simulink model "land_V0"  (R2023b)
settings: Solver=ode4  StartTime=0.0  StopTime=150  FixedStep=0.001  RelTol=1e-3
values from neighbouring files (symbols this model uses):
  a0 = 340.294    [basedata.m]    (also in basedata.mat; control_design.mat; landing_init.m; landing_plan.mat)
  b_ref = 2.0    (= 2)    [basedata.m]    (also in basedata.mat; control_design.mat; landing_init.m; landing_plan.mat)
  c_gear = [0.8e4, 1.4e4, 1.4e4]    [basedata.m]    (also in basedata.mat = [8000 14000 14000]; control_design.mat = [8000 14000 14000]; landing_init.m; landing_plan.mat = [8000 14000 14000])
  c_lat = [1.4e4, 2.2e4, 2.2e4]    [basedata.m]    (also in basedata.mat = [14000 22000 22000]; control_design.mat = [14000 22000 22000]; landing_init.m; landing_plan.mat = [14000 22000 22000])
  c_ref = 0.9    [basedata.m]    (also in basedata.mat; control_design.mat; landing_init.m; landing_plan.mat)
  c_roll = [0.020, 0.018, 0.018]    [basedata.m]    (also in basedata.mat = [0.02 0.018 0.018]; control_design.mat = [0.02 0.018 0.018]; landing_init.m; landing_plan.mat = [0.02 0.018 0.018])
  CD0 = 0.045    [basedata.m]    (also in basedata.mat; canshujisuan.m; control_design.mat; landing_init.m)
  CL0 = 0.083    [basedata.m]    (also in basedata.mat; control_design.mat; landing_init.m; landing_plan.mat)
  CLa = 3.80    (= 3.8)    [basedata.m]    (also in basedata.mat; canshujisuan.m = 2.5; control_design.mat; landing_init.m)
  Clb = -0.08    [basedata.m]    (also in basedata.mat; control_design.mat; landing_init.m; landing_plan.mat)
  Clda = -0.20    (= -0.2)    [basedata.m]    (also in basedata.mat; control_design.mat; landing_init.m; landing_plan.mat)
  CLde = 0.28    [basedata.m]    (also in basedata.mat; control_design.mat; landing_init.m; landing_plan.mat)
  Clp = -0.70    (= -0.7)    [basedata.m]    (also in basedata.mat; control_design.mat; landing_init.m; landing_plan.mat)
  CLq = 4.50    (= 4.5)    [basedata.m]    (also in basedata.mat; canshujisuan.m = 3; control_design.mat; landing_init.m)
  Clr = 0.08    [basedata.m]    (also in basedata.mat; control_design.mat; landing_init.m; landing_plan.mat)
  Cm0 = 0.060    (= 0.06)    [basedata.m]    (also in basedata.mat; control_design.mat; landing_init.m; landing_plan.mat)
  Cma = -0.80    (= -0.8)    [basedata.m]    (also in basedata.mat; control_design.mat; landing_init.m; landing_plan.mat)
  Cmde = -0.90    (= -0.9)    [basedata.m]    (also in basedata.mat; control_design.mat; landing_init.m; landing_plan.mat)
  Cmq = -18.0    (= -18)    [basedata.m]    (also in basedata.mat; control_design.mat; landing_init.m; landing_plan.mat)
  Cnb = 0.25    [basedata.m]    (also in basedata.mat; control_design.mat; landing_init.m; landing_plan.mat)
  Cndr = -0.15    [basedata.m]    (also in basedata.mat; control_design.mat; landing_init.m; landing_plan.mat)
  Cnp = -0.04    [basedata.m]    (also in basedata.mat; control_design.mat; landing_init.m; landing_plan.mat)
  Cnr = -0.45    [basedata.m]    (also in basedata.mat; control_design.mat; landing_init.m; landing_plan.mat)
  CSb = -0.70    (= -0.7)    [basedata.m]    (also in basedata.mat; control_design.mat; landing_init.m; landing_plan.mat)
  CSdr = 0.18    [basedata.m]    (also in basedata.mat; control_design.mat; landing_init.m; landing_plan.mat)
  CSr = 0.12    [basedata.m]    (also in basedata.mat; control_design.mat; landing_init.m; landing_plan.mat)
  D = 0.5 * rho0 * V^2 * S_ref * CD_current    [canshujisuan.m]
  D0 = 1400    [basedata.m]    (also in basedata.mat; control_design.mat = 800; landing.m; landing_init.m)
  da_max = 25    [basedata.m]    (also in basedata.mat; control_design.mat; landing_init.m; landing_plan.mat)
  da_min = -da_max    (= -25)    [basedata.m]    (also in basedata.mat; control_design.mat; landing_init.m; landing_plan.mat)
  de_max = 25    [basedata.m]    (also in basedata.mat; control_design.mat; landing_init.m; landing_plan.mat)
  de_min = -de_max    (= -25)    [basedata.m]    (also in basedata.mat; control_design.mat; landing_init.m; landing_plan.mat)
  DH = pi / 180    (= 0.0174532925199)    [basedata.m]    (also in basedata.mat; control_design.mat; landing_init.m; landing_plan.mat)
  dr_max = 25    [basedata.m]    (also in basedata.mat; control_design.mat; landing_init.m; landing_plan.mat)
  dr_min = -dr_max    (= -25)    [basedata.m]    (also in basedata.mat; control_design.mat; landing_init.m; landing_plan.mat)
  g = 9.80665    [basedata.m]    (also in basedata.mat; canshujisuan.m; control_design.mat; landing_init.m)
  gamma1 = -0.125844364415    [basedata.mat]    (also in landing_trajectory.m = asin(max(min(gamma1_arg, 1), -1)); landingplan.mat)
  gamma2 = -0.0261780104712    [basedata.mat]    (also in landing_trajectory.m = -0.0261799387799; landingplan.mat = 0.0261780104712)
  ground_z = 0.0    (= 0)    [basedata.m]    (also in basedata.mat; control_design.mat; landing_init.m; landing_plan.mat)
  HD = 180 / pi    (= 57.2957795131)    [basedata.m]    (also in basedata.mat; control_design.mat; landing_init.m; landing_plan.mat)
  I = [ Ixx, -Ixy, -Ixz ... (first row only)    [basedata.m]    (also in basedata.mat = [120  0  0; 0  480  0; 0  0  520]; control_design.mat = [120  0  0; 0  480  0; 0  0  520]; landing_init.m; landing_plan.mat = [120  0  0; 0  480  0; 0  0  520])
  K = 0.12    [basedata.m]    (also in basedata.mat; canshujisuan.m = 0.08; control_design.mat; landing_init.m)
  K_alpha = 7.5375    [basedata.mat]    (also in control_design.m = (((wd_pitch^2)-a24))/(2*kesi_pitch*wd_pitch); control_design.mat; controller.m = 5; landingplan.mat)
  k_gear = [1.0e5, 3.0e5, 3.0e5]    [basedata.m]    (also in basedata.mat = [100000 300000 300000]; control_design.mat = [100000 300000 300000]; landing_init.m; landing_plan.mat = [100000 300000 300000])
  Kn_pitch = -0.120095403309    [basedata.mat]    (also in control_design.m = -(2.2*g*(wd_pitch)^2)/(Tr*(((wd_pitch)^2)-a24)*V_control*a34; control_design.mat; controller.m = (2.2*wd^2*g)/(Tr*(wd^2-a24)*V_test*a34); landingplan.mat)
  Kw_pitch = -0.483749055178    [basedata.mat]    (also in control_design.m = -2*kesi_pitch*wd_pitch/a25; control_design.mat; controller.m = -(2*zeta*wd) / a25; landingplan.mat)
  m = 600.0    (= 600)    [basedata.m]    (also in basedata.mat; canshujisuan.m; control_design.mat; landing_init.m)
  mu_brake = [0.0, 0.55, 0.55]    [basedata.m]    (also in basedata.mat = [0 0.55 0.55]; control_design.mat = [0 0.55 0.55]; landing_init.m; landing_plan.mat = [0 0.55 0.55])
  phi0 = 0    [control_design.mat]    (also in landing.m; landing_init.m; landing_init.mat; landing_plan.mat)
  psi0 = 0    [control_design.mat]    (also in landing.m; landing_init.m; landing_init.mat; landing_plan.mat)
  r_left_b = r_gear_b(:,2)    [basedata.m]    (also in basedata.mat = [-0.333333333333 -0.8 0.65]; control_design.mat = [-0.333333333333 -0.8 0.65]; landing_init.m; landing_plan.mat = [-0.333333333333 -0.8 0.65])
  r_nose_b = r_gear_b(:,1)    [basedata.m]    (also in basedata.mat = [2 0 0.65]; control_design.mat = [2 0 0.65]; landing_init.m; landing_plan.mat = [2 0 0.65])
  r_right_b = r_gear_b(:,3)    [basedata.m]    (also in basedata.mat = [-0.333333333333 0.8 0.65]; control_design.mat = [-0.333333333333 0.8 0.65]; landing_init.m; landing_plan.mat = [-0.333333333333 0.8 0.65])
  rho0 = 1.225    [basedata.m]    (also in basedata.mat; canshujisuan.m; control_design.mat; landing_init.m)
  S_ref = 1.2    [basedata.m]    (also in basedata.mat; canshujisuan.m; control_design.mat; landing_init.m)
  theta0 = 0    [control_design.mat]    (also in landing.m; landing_init.m; landing_init.mat = 0.0523598775598; landing_plan.mat = 0.0523560209424)
  u0_b = 0    [control_design.mat]    (also in landing.m = 128; landing_init.m = 128; landing_init.mat = 100; landing_plan.mat = 128)
  v0_b = 0    [control_design.mat]    (also in landing.m; landing_init.m; landing_init.mat; landing_plan.mat)
  v_eps = 0.20    (= 0.2)    [basedata.m]    (also in basedata.mat; control_design.mat; landing_init.m; landing_plan.mat)
  V_min = 3    [control_design.mat]    (also in landing.m; landing_init.m; landing_plan.mat; landingplan.mat)
  w0_b = 0    [control_design.mat]    (also in landing.m; landing_init.m; landing_init.mat; landing_plan.mat)
  wheel_radius = 0.18    [basedata.m]    (also in basedata.mat; control_design.mat; landing_init.m; landing_plan.mat)
  WOW_on = 0.000    (= 0)    [basedata.m]    (also in basedata.mat; control_design.mat; landing_init.m; landing_plan.mat)
  Xg0 = 0    [control_design.mat]    (also in landing.m = -12000; landing_init.m = -12000; landing_init.mat = -8000; landing_plan.mat = -12000)
  Yg0 = 3    [control_design.mat]    (also in landing.m = 0; landing_init.m = 0; landing_init.mat = 0; landing_plan.mat = 0)
  Zg0 = ground_z - wheel_radius - r_gear_b(3,1) + static_deflection    [basedata.m]    (also in basedata.mat = -0.8215943; control_design.mat = -0.8215943; landing.m = -1000; landing_init.m = -1000)
undefined symbols (not defined in the file or in its folder): I_xz, I_yz, Ix_Iy, Iy_Iz, Iz_Ix
libraries: simulink x37, matrix_library x19
(part 3 of 3)

== system land_V0/6DOF-MODEL/动力学/起落架模型/起落架三轮质心在地系下位置 ==
  Add : Sum
  Add1 : Sum
  Add2 : Sum
  Constant : Constant  Value=r_nose_b
  Constant1 : Constant  Value=r_left_b
  Constant2 : Constant  Value=r_right_b
  MATLAB Function : MATLAB Function  TreatAsAtomicUnit=on
  Matrix Multiply : Product  Multiplication=Matrix(*)
  Matrix Multiply1 : Product  Multiplication=Matrix(*)
  Matrix Multiply2 : Product  Multiplication=Matrix(*)
  Mux : Mux  Inputs=3
  Scope : Scope
  Scope1 : Scope
  Scope2 : Scope
  Selector : Selector  InputPortWidth=3  IndexOptions=Index vector (dialog)  Indices=2  OutputSizes=1
  Transpose : matrix_library/Transpose
  Nose_pos_g : Outport
  Left_pos_g : Outport  Port=2
  Right_pos_g : Outport  Port=3
  tag scope: Left_pos_g=global, Nose_position_g=global, Right_pos_g=global
  wires:
  Constant1/1 -> Matrix Multiply1/2
  Transpose/1 -> Matrix Multiply2/1, Matrix Multiply1/1, Matrix Multiply/1
  [psi_eular] -> MATLAB Function/3(psi)
  [phi_eular] -> MATLAB Function/1(phi), Scope2/1
  Constant2/1 -> Matrix Multiply2/2
  Matrix Multiply1/1 -> Add1/2
  Constant/1 -> Matrix Multiply/2
  [theta_eular] -> MATLAB Function/2(theta)
  MATLAB Function/1(R_bg) -> Transpose/1
  Matrix Multiply/1 -> Add/2
  Matrix Multiply2/1 -> Add2/2
  [Z_positon] -> Mux/3
  [Y_positon] -> Scope1/1, Mux/2
  [X_positon] -> Mux/1
  Mux/1 -> Add/1, Add1/1, Add2/1
  Add/1 -> Selector/1, Nose_pos_g/1, [Nose_position_g]
  Add1/1 -> Left_pos_g/1, [Left_pos_g]
  Add2/1 -> Right_pos_g/1, [Right_pos_g]
  Selector/1 -> Scope/1

== system land_V0/6DOF-MODEL/动力学/起落架模型/轮胎压缩量计算 ==
  Nose_pos_g : Inport
  Left_pos_g : Inport  Port=2
  Right_pos_g : Inport  Port=3
  Constant : Constant  Value=wheel_radius
  Constant1 : Constant  Value=ground_z
  Constant2 : Constant  Value=0
  Constant4 : Constant
  Saturation : Saturate  UpperLimit=wheel_radius  LowerLimit=0
  Saturation1 : Saturate  UpperLimit=wheel_radius  LowerLimit=0
  Saturation2 : Saturate  UpperLimit=wheel_radius  LowerLimit=0
  Scope : Scope
  Scope1 : Scope
  Selector : Selector  InputPortWidth=3  IndexOptions=Index vector (dialog)  Indices=3  OutputSizes=1
  Selector1 : Selector  InputPortWidth=3  IndexOptions=Index vector (dialog)  Indices=3  OutputSizes=1
  Selector2 : Selector  InputPortWidth=3  IndexOptions=Index vector (dialog)  Indices=3  OutputSizes=1
  Subtract{,1..5} (6 alike) : Sum  Inputs=+-
  Switch3 : Switch  Criteria=u2 > Threshold  Threshold=WOW_on  SaturateOnIntegerOverflow=off  InputSameDT=off
  Switch4 : Switch  Criteria=u2 > Threshold  Threshold=WOW_on  SaturateOnIntegerOverflow=off  InputSameDT=off
  Switch5 : Switch  Criteria=u2 > Threshold  Threshold=WOW_on  SaturateOnIntegerOverflow=off  InputSameDT=off
  delta_nose : Outport
  delta_left : Outport  Port=2
  delta_right : Outport  Port=3
  tag scope: contact_left=global, contact_nose=global, contact_right=global, delta_left=global, delta_nose=global, delta_right=global
  wires:
  Nose_pos_g/1 -> Selector/1
  Left_pos_g/1 -> Selector1/1
  Right_pos_g/1 -> Selector2/1
  Subtract/1 -> Subtract3/2
  Subtract1/1 -> Subtract4/2
  Subtract2/1 -> Subtract5/2
  Constant/1 -> Subtract5/1, Subtract4/1, Subtract3/1
  Saturation/1 -> Scope/1, delta_nose/1, [delta_nose]
  Saturation1/1 -> [delta_left], delta_left/1, Scope1/1
  Saturation2/1 -> [delta_right], delta_right/1
  Subtract3/1 -> Switch3/2, Saturation/1
  Subtract4/1 -> Switch4/2, Saturation1/1
  Subtract5/1 -> Switch5/2, Saturation2/1
  Constant2/1 -> Switch3/3, Switch5/3, Switch4/3
  Constant4/1 -> Switch5/1, Switch4/1, Switch3/1
  Switch3/1 -> [contact_nose]
  Switch5/1 -> [contact_right]
  Switch4/1 -> [contact_left]
  Constant1/1 -> Subtract/1, Subtract1/1, Subtract2/1
  Selector/1 -> Subtract/2
  Selector1/1 -> Subtract1/2
  Selector2/1 -> Subtract2/2

== system land_V0/controller1/1_Pitch_Ctrl/567三回路控制/Subsystem ==
  q : Inport
  Integrator : Integrator
  Product : Product
  Subsystem : Subsystem
  Sum : Sum  Inputs=|+-
  alpha(伪攻角) : Outport
  wires:
  q/1 -> Sum/1
  Sum/1 -> Integrator/1
  Integrator/1 -> Product/1, alpha(伪攻角)/1
  Product/1 -> Sum/2
  Subsystem/1(a34) -> Product/2

== system land_V0/6DOF-MODEL/动力学/起落架模型/三轮在地系下的力/摩擦圆限幅 ==
  N_nose : Inport
  N_left : Inport  Port=2
  N_right : Inport  Port=3
  F_long_nose : Inport  Port=4
  F_long_left : Inport  Port=5
  F_long_right : Inport  Port=6
  F_lat_nose : Inport  Port=7
  F_lat_left : Inport  Port=8
  F_lat_right : Inport  Port=9
  主轮摩擦圆限幅右 : MATLAB Function  TreatAsAtomicUnit=on
  主轮摩擦圆限幅左 : MATLAB Function  TreatAsAtomicUnit=on
  前轮摩擦圆限幅 : MATLAB Function  TreatAsAtomicUnit=on
  F_long_nose_out : Outport
  F_long_left_out : Outport  Port=2
  F_long_right_out : Outport  Port=3
  F_lat__nose_out : Outport  Port=4
  F_lat_left_out : Outport  Port=5
  F_lat_right_out : Outport  Port=6
  wires:
  前轮摩擦圆限幅/1(F_long_out) -> F_long_nose_out/1
  前轮摩擦圆限幅/2(F_lat_out) -> F_lat__nose_out/1
  主轮摩擦圆限幅左/2(F_lat_out) -> F_lat_left_out/1
  主轮摩擦圆限幅左/1(F_long_out) -> F_long_left_out/1
  主轮摩擦圆限幅右/2(F_lat_out) -> F_lat_right_out/1
  主轮摩擦圆限幅右/1(F_long_out) -> F_long_right_out/1
  N_nose/1 -> 前轮摩擦圆限幅/1(N)
  F_long_nose/1 -> 前轮摩擦圆限幅/2(F_long)
  F_lat_nose/1 -> 前轮摩擦圆限幅/3(F_lat)
  F_long_left/1 -> 主轮摩擦圆限幅左/2(F_long)
  N_left/1 -> 主轮摩擦圆限幅左/1(N)
  F_lat_right/1 -> 主轮摩擦圆限幅右/3(F_lat)
  F_lat_left/1 -> 主轮摩擦圆限幅左/3(F_lat)
  F_long_right/1 -> 主轮摩擦圆限幅右/2(F_long)
  N_right/1 -> 主轮摩擦圆限幅右/1(N)

== system land_V0/6DOF-MODEL/动力学/起落架模型/侧向力/Subsystem ==
  delt-s(H) : Inport
  Constant : Constant  Value=0
  Constant1 : Constant  Value=0
  Constant2 : Constant  Value=0
  Constant3 : Constant
  Cos : Trigonometry  Operator=cos
  Gain : Gain  Gain=-1
  Hermitian Transpose{,1..3} (4 alike) : matrix_library/Hermitian Transpose
  MATLAB Function : MATLAB Function  TreatAsAtomicUnit=on
  Matrix Multiply : Product  Multiplication=Matrix(*)
  Matrix Multiply1 : Product  Multiplication=Matrix(*)
  Matrix Multiply2 : Product  Multiplication=Matrix(*)
  Mux : Mux  Inputs=3
  Mux1 : Mux  Inputs=3
  Reshape : Reshape  OutputDimensionality=Column vector (2-D)
  Reshape1 : Reshape  OutputDimensionality=Column vector (2-D)
  Sin : Trigonometry
  主轮侧向方向向量 : MATLAB Function  TreatAsAtomicUnit=on
  前轮侧向向量 : MATLAB Function  TreatAsAtomicUnit=on
  V_lat_nose : Outport
  V_lat_left : Outport  Port=2
  V_lat_right : Outport  Port=3
  tag scope: V_lat_left=global, V_lat_nose=global, V_lat_right=global, e_g_lat_main=global, e_g_lat_nose=global
  wires:
  MATLAB Function/1(R_bg) -> Hermitian Transpose/1
  [phi_eular] -> MATLAB Function/1(phi)
  Hermitian Transpose/1 -> 主轮侧向方向向量/1(Cbg), 前轮侧向向量/1(Cbg)
  Mux/1 -> Reshape/1
  Constant1/1 -> Mux1/1
  Mux1/1 -> Reshape1/1
  [V_nose_g] -> Hermitian Transpose1/1
  前轮侧向向量/1(eg_lat) -> [e_g_lat_nose], Matrix Multiply/2
  Hermitian Transpose1/1 -> Matrix Multiply/1
  [V_left_g] -> Hermitian Transpose2/1
  [V_right_g] -> Hermitian Transpose3/1
  主轮侧向方向向量/1(eg_lat) -> Matrix Multiply2/2, Matrix Multiply1/2, [e_g_lat_main]
  Hermitian Transpose3/1 -> Matrix Multiply1/1
  Hermitian Transpose2/1 -> Matrix Multiply2/1
  Matrix Multiply/1 -> V_lat_nose/1, [V_lat_nose]
  Matrix Multiply2/1 -> V_lat_left/1, [V_lat_left]
  Matrix Multiply1/1 -> V_lat_right/1, [V_lat_right]
  Sin/1 -> Gain/1
  Gain/1 -> Mux/1
  delt-s(H)/1 -> Sin/1, Cos/1
  [theta_eular] -> MATLAB Function/2(theta)
  [psi_eular] -> MATLAB Function/3(psi)
  Reshape/1 -> 前轮侧向向量/2(eb_lat)
  Reshape1/1 -> 主轮侧向方向向量/2(eb_lat)
  Cos/1 -> Mux/2
  Constant/1 -> Mux/3
  Constant3/1 -> Mux1/2
  Constant2/1 -> Mux1/3

== system land_V0/6DOF-MODEL/动力学/起落架模型/侧向力/Subsystem1 ==
  In1 : Inport
  Constant5 : Constant  Value=0
  Switch : Switch  Criteria=u2 > Threshold  SaturateOnIntegerOverflow=off  InputSameDT=off
  F_lat_left : Outport
  wires:
  In1/1 -> Switch/1
  Constant5/1 -> Switch/3
  Switch/1 -> F_lat_left/1
  [contact_left] -> Switch/2

== system land_V0/6DOF-MODEL/动力学/起落架模型/侧向力/Subsystem2 ==
  In1 : Inport
  Constant5 : Constant  Value=0
  Switch : Switch  Criteria=u2 > Threshold  SaturateOnIntegerOverflow=off  InputSameDT=off
  F_lat_nose : Outport
  wires:
  In1/1 -> Switch/1
  Constant5/1 -> Switch/3
  Switch/1 -> F_lat_nose/1
  [contact_nose] -> Switch/2

== system land_V0/6DOF-MODEL/动力学/起落架模型/侧向力/Subsystem3 ==
  In1 : Inport
  Constant5 : Constant  Value=0
  Switch : Switch  Criteria=u2 > Threshold  SaturateOnIntegerOverflow=off  InputSameDT=off
  F_lat_right : Outport
  wires:
  [contact_right] -> Switch/2
  Switch/1 -> F_lat_right/1
  Constant5/1 -> Switch/3
  In1/1 -> Switch/1

== system land_V0/6DOF-MODEL/动力学/起落架模型/法向支反力/Subsystem ==
  In1 : Inport
  Constant5 : Constant  Value=0
  Switch : Switch  Criteria=u2 > Threshold  SaturateOnIntegerOverflow=off  InputSameDT=off
  N_nose : Outport
  wires:
  In1/1 -> Switch/1
  Constant5/1 -> Switch/3
  Switch/1 -> N_nose/1
  [contact_nose] -> Switch/2

== system land_V0/6DOF-MODEL/动力学/起落架模型/法向支反力/Subsystem1 ==
  In1 : Inport
  Constant5 : Constant  Value=0
  Switch : Switch  Criteria=u2 > Threshold  SaturateOnIntegerOverflow=off  InputSameDT=off
  N_left : Outport
  wires:
  [contact_left] -> Switch/2
  Switch/1 -> N_left/1
  Constant5/1 -> Switch/3
  In1/1 -> Switch/1

== system land_V0/6DOF-MODEL/动力学/起落架模型/法向支反力/Subsystem2 ==
  In1 : Inport
  Constant5 : Constant  Value=0
  Switch : Switch  Criteria=u2 > Threshold  SaturateOnIntegerOverflow=off  InputSameDT=off
  N_right : Outport
  wires:
  In1/1 -> Switch/1
  Constant5/1 -> Switch/3
  Switch/1 -> N_right/1
  [contact_right] -> Switch/2

== system land_V0/6DOF-MODEL/动力学/起落架模型/纵向力/Subsystem ==
  delt-s(H) : Inport
  Constant : Constant  Value=0
  Constant1 : Constant
  Constant2 : Constant  Value=0
  Constant3 : Constant  Value=0
  Cos : Trigonometry  Operator=cos
  Hermitian Transpose{,1..3} (4 alike) : matrix_library/Hermitian Transpose
  MATLAB Function : MATLAB Function  TreatAsAtomicUnit=on
  Matrix Multiply : Product  Multiplication=Matrix(*)
  Matrix Multiply1 : Product  Multiplication=Matrix(*)
  Matrix Multiply2 : Product  Multiplication=Matrix(*)
  Mux : Mux  Inputs=3
  Mux1 : Mux  Inputs=3
  Reshape : Reshape  OutputDimensionality=Column vector (2-D)
  Reshape1 : Reshape  OutputDimensionality=Column vector (2-D)
  Sin : Trigonometry
  主轮滚动方向向量 : MATLAB Function  TreatAsAtomicUnit=on
  前轮滚动方向向量 : MATLAB Function  TreatAsAtomicUnit=on
  V_long_nose : Outport
  V_long_left : Outport  Port=2
  V_long_right : Outport  Port=3
  tag scope: V_long_left=global, V_long_nose=global, V_long_right=global, e_g_long_main=global, e_g_long_nose=global
  wires:
  MATLAB Function/1(R_bg) -> Hermitian Transpose/1
  [phi_eular] -> MATLAB Function/1(phi)
  Hermitian Transpose/1 -> 主轮滚动方向向量/1(Cbg), 前轮滚动方向向量/1(Cbg)
  delt-s(H)/1 -> Cos/1, Sin/1
  Cos/1 -> Mux/1
  Mux/1 -> Reshape/1
  Constant1/1 -> Mux1/1
  Constant2/1 -> Mux1/2
  Constant3/1 -> Mux1/3
  Mux1/1 -> Reshape1/1
  [V_nose_g] -> Hermitian Transpose1/1
  前轮滚动方向向量/1(eg_long) -> [e_g_long_nose], Matrix Multiply/2
  Hermitian Transpose1/1 -> Matrix Multiply/1
  [V_left_g] -> Hermitian Transpose2/1
  [V_right_g] -> Hermitian Transpose3/1
  主轮滚动方向向量/1(eg_long) -> Matrix Multiply1/2, Matrix Multiply2/2, [e_g_long_main]
  Hermitian Transpose3/1 -> Matrix Multiply1/1
  Hermitian Transpose2/1 -> Matrix Multiply2/1
  Matrix Multiply/1 -> V_long_nose/1, [V_long_nose]
  Matrix Multiply2/1 -> V_long_left/1, [V_long_left]
  Matrix Multiply1/1 -> V_long_right/1, [V_long_right]
  [theta_eular] -> MATLAB Function/2(theta)
  [psi_eular] -> MATLAB Function/3(psi)
  Reshape/1 -> 前轮滚动方向向量/2(eb_long)
  Reshape1/1 -> 主轮滚动方向向量/2(eb_long)
  Sin/1 -> Mux/2
  Constant/1 -> Mux/3

== system land_V0/6DOF-MODEL/动力学/起落架模型/纵向力/Subsystem1 ==
  V_long_nose : Inport
  V_long_left : Inport  Port=2
  V_long_right : Inport  Port=3
  u_brake : Inport  Port=4
  Add : Sum
  Add1 : Sum
  Add2 : Sum
  Constant : Constant  Value=v_eps
  Divide : Product  Inputs=*/
  Divide1 : Product  Inputs=*/
  Divide2 : Product  Inputs=*/
  Subsystem : Subsystem
  Subsystem1 : Subsystem
  Subsystem2 : Subsystem
  Subsystem3 : Subsystem
  Subsystem4 : Subsystem
  Tanh : Trigonometry  Operator=tanh
  Tanh1 : Trigonometry  Operator=tanh
  Tanh2 : Trigonometry  Operator=tanh
  F_long_nose : Outport
  F_long_left : Outport  Port=2
  F_long_right : Outport  Port=3
  wires:
  Divide1/1 -> Tanh1/1
  V_long_right/1 -> Divide2/1
  Divide2/1 -> Tanh2/1
  Constant/1 -> Divide1/2, Divide/2, Divide2/2
  Divide/1 -> Tanh/1
  V_long_left/1 -> Divide1/1
  V_long_nose/1 -> Divide/1
  u_brake/1 -> Subsystem/4(u_brake)
  Subsystem1/1(F_roll_nose) -> Add/1
  Subsystem1/2(F_roll_left) -> Add1/1
  Subsystem1/3(F_roll_right) -> Add2/1
  Subsystem/1(F_brake_nose) -> Add/2
  Subsystem/2(F_brake_left) -> Add1/2
  Subsystem/3(F_brake_right) -> Add2/2
  Tanh/1 -> Subsystem1/1(sig_nose), Subsystem/1(sig_nose)
  Tanh1/1 -> Subsystem1/2(sig_left), Subsystem/2(sig_left)
  Tanh2/1 -> Subsystem1/3(sig_right), Subsystem/3(sig_right)
  Add/1 -> Subsystem2/1(In1)
  Add1/1 -> Subsystem3/1(In1)
  Add2/1 -> Subsystem4/1(In1)
  Subsystem2/1(F_long_nose) -> F_long_nose/1
  Subsystem3/1(F_long_left) -> F_long_left/1
  Subsystem4/1(F_long_right) -> F_long_right/1

== system land_V0/controller1/1_Pitch_Ctrl/567三回路控制/Subsystem/Subsystem ==
  Add : Sum
  Constant : Constant  Value=CLa
  Constant1 : Constant  Value=S_ref
  Constant2 : Constant  Value=m
  Constant3 : Constant  Value=D0
  Divide : Product  Inputs=*/
  Product : Product  Inputs=3
  Product1 : Product
  a34 : Outport
  wires:
  Constant/1 -> Product/1
  Constant1/1 -> Product/2
  [qc] -> Product/3
  Divide/1 -> a34/1
  [Va_safe] -> Product1/2
  Constant2/1 -> Product1/1
  Product1/1 -> Divide/2
  Constant3/1 -> Add/1
  Product/1 -> Add/2
  Add/1 -> Divide/1

== system land_V0/6DOF-MODEL/动力学/起落架模型/纵向力/Subsystem1/Subsystem ==
  sig_nose : Inport
  sig_left : Inport  Port=2
  sig_right : Inport  Port=3
  u_brake : Inport  Port=4
  Constant2 : Constant  Value=mu_brake
  Demux1 : Demux  Outputs=3
  Gain3 : Gain  Gain=-1
  Product3 : Product  Inputs=4
  Product4 : Product  Inputs=4
  Product5 : Product  Inputs=4
  F_brake_nose : Outport
  F_brake_left : Outport  Port=2
  F_brake_right : Outport  Port=3
  wires:
  Demux1/2 -> Product4/4
  Gain3/1 -> Product3/3, Product4/3, Product5/3
  Demux1/3 -> Product5/4
  u_brake/1 -> Gain3/1
  Constant2/1 -> Demux1/1
  Demux1/1 -> Product3/4
  sig_right/1 -> Product5/2
  Product3/1 -> F_brake_nose/1
  Product5/1 -> F_brake_right/1
  Product4/1 -> F_brake_left/1
  sig_nose/1 -> Product3/2
  sig_left/1 -> Product4/2
  [N_nose] -> Product3/1
  [N_left] -> Product4/1
  [N_right] -> Product5/1

== system land_V0/6DOF-MODEL/动力学/起落架模型/纵向力/Subsystem1/Subsystem1 ==
  sig_nose : Inport
  sig_left : Inport  Port=2
  sig_right : Inport  Port=3
  Constant1 : Constant  Value=c_roll
  Demux : Demux  Outputs=3
  Gain : Gain  Gain=-1
  Gain1 : Gain  Gain=-1
  Gain2 : Gain  Gain=-1
  Product : Product  Inputs=3
  Product1 : Product  Inputs=3
  Product2 : Product  Inputs=3
  F_roll_nose : Outport
  F_roll_left : Outport  Port=2
  F_roll_right : Outport  Port=3
  wires:
  sig_left/1 -> Product1/3
  Demux/2 -> Product1/2
  Gain1/1 -> F_roll_left/1
  Constant1/1 -> Demux/1
  Product1/1 -> Gain1/1
  Demux/1 -> Product/2
  Demux/3 -> Product2/2
  Gain/1 -> F_roll_nose/1
  Product/1 -> Gain/1
  Product2/1 -> Gain2/1
  sig_right/1 -> Product2/3
  Gain2/1 -> F_roll_right/1
  sig_nose/1 -> Product/3
  [N_nose] -> Product/1
  [N_left] -> Product1/1
  [N_right] -> Product2/1

== system land_V0/6DOF-MODEL/动力学/起落架模型/纵向力/Subsystem1/Subsystem2 ==
  In1 : Inport
  Constant5 : Constant  Value=0
  Switch : Switch  Criteria=u2 > Threshold  SaturateOnIntegerOverflow=off  InputSameDT=off
  F_long_nose : Outport
  wires:
  In1/1 -> Switch/1
  Constant5/1 -> Switch/3
  Switch/1 -> F_long_nose/1
  [contact_nose] -> Switch/2

== system land_V0/6DOF-MODEL/动力学/起落架模型/纵向力/Subsystem1/Subsystem3 ==
  In1 : Inport
  Constant5 : Constant  Value=0
  Switch : Switch  Criteria=u2 > Threshold  SaturateOnIntegerOverflow=off  InputSameDT=off
  F_long_left : Outport
  wires:
  In1/1 -> Switch/1
  Constant5/1 -> Switch/3
  Switch/1 -> F_long_left/1
  [contact_left] -> Switch/2

== system land_V0/6DOF-MODEL/动力学/起落架模型/纵向力/Subsystem1/Subsystem4 ==
  In1 : Inport
  Constant5 : Constant  Value=0
  Switch : Switch  Criteria=u2 > Threshold  SaturateOnIntegerOverflow=off  InputSameDT=off
  F_long_right : Outport
  wires:
  [contact_right] -> Switch/2
  Switch/1 -> F_long_right/1
  Constant5/1 -> Switch/3
  In1/1 -> Switch/1

== matlab function land_V0/Guidance/4_拉平制导/MATLAB Function ==
  settings: updateMethod=DISCRETE  sampleTime=0.001
  data: Flight_Phase input; H_cmd output; t input
function H_cmd = flare_H_cmd(Flight_Phase, t)
%#codegen

FLARE_PHASE = 11;

H0        = 20.0;   % 拉平起始指令高度，应等于浅下滑段末端高度
T_flare   = 6.0;    % 拉平时间常数
V_sink_td = 0.5;    % 接地下沉率，若想最终更水平可改小

persistent t_enter last_phase

if isempty(t_enter)
    t_enter = 0.0;
    last_phase = uint8(0);
end

if Flight_Phase == FLARE_PHASE && last_phase ~= FLARE_PHASE
    t_enter = t;
end

if Flight_Phase == FLARE_PHASE
    tau = max(t - t_enter, 0.0);

    H_raw = (H0 + V_sink_td*T_flare) * exp(-tau/T_flare) ...
            - V_sink_td*T_flare;

    H_cmd = max(H_raw, 0.0);
else
    H_cmd = H0;
end

last_phase = Flight_Phase;

== matlab function land_V0/Guidance/3_空中制导/gamma切换/MATLAB Function ==
  data: X input; gamma_cmd output
function gamma_cmd = round_gamma_cmd(X)
%#codegen
% 圆拉平段下滑角指令
% X: 当前地面坐标 X, m
% gamma_cmd: 下滑角指令, rad, 下降为负

X_B = -4048.3;
X_C = -3253.6;
X_R = -3044.2;
R   = 8000.0;

X_use = X;

if X_use < X_B
    X_use = X_B;
elseif X_use > X_C
    X_use = X_C;
end

dx = X_use - X_R;
rad = R^2 - dx^2;

if rad < 1e-6
    rad = 1e-6;
end

dH_dX = dx / sqrt(rad);
gamma_cmd = atan(dH_dX);

== matlab function land_V0/6DOF-MODEL/AERO-PARAMETER/atmosphere/MATLAB Function ==
  data: phi input; R_bg output; theta input; psi input
function R_bg = ground2body(phi, theta, psi)
T1 = [cos(psi), sin(psi), 0;
     -sin(psi), cos(psi), 0;
      0, 0, 1];
T2 = [cos(theta), 0, -sin(theta);
       0, 1, 0;
      sin(theta), 0, cos(theta)];
T3 = [1, 0, 0;
      0, cos(phi), sin(phi);
      0, -sin(phi), cos(phi)];
R_bg = T3 * T2 * T1;

== matlab function land_V0/6DOF-MODEL/动力学/Subsystem3/MATLAB Function ==
  data: phi input; R_bg output; theta input; psi input
function R_bg = ground2body(phi, theta, psi)
T1 = [cos(psi), sin(psi), 0;
     -sin(psi), cos(psi), 0;
      0, 0, 1];
T2 = [cos(theta), 0, -sin(theta);
       0, 1, 0;
      sin(theta), 0, cos(theta)];
T3 = [1, 0, 0;
      0, cos(phi), sin(phi);
      0, -sin(phi), cos(phi)];
R_bg = T3 * T2 * T1;

== matlab function land_V0/6DOF-MODEL/动力学/dynamics EQ/MATLAB Function ==
  data: alpha input; R_bwind output; beta input
function R_bwind = wind2body(alpha, beta)
T1 = [cos(alpha), 0, sin(alpha);
       0, 1, 0;
       -sin(alpha), 0, cos(alpha)];
T2 = [cos(beta), sin(beta), 0;
       -sin(beta), cos(beta), 0;
       0, 0, 1];
R_wind_b = T2*T1;
R_bwind = R_wind_b';

== matlab function land_V0/controller1/4_Power&V_Ctrl/MATLAB Function ==
  data: Vel_g input; dv_err output; axyz input
function dv_err = dv_cal(Vel_g,axyz)
%#codegen

% k_theta = Att_g(1)*pi/180;
% psi = Att_g(2)*pi/180;
% gama = Att_g(3)*pi/180;
% 
% Cg_b = Mx(gama)*Mz(k_theta)*My(psi);
% Cb_g = Cg_b';
vx = Vel_g(1);
vy = Vel_g(2);
vz = Vel_g(3);

ax = axyz(1);
ay = axyz(2);
az = axyz(3);

dv_err = (vx*ax + vy*ay + vz*az)/sqrt(vx^2 + vy^2 + vz^2);
% dv_err = (vx*ax + vz*az)/sqrt(vx^2 + vz^2);
if isnan(dv_err) == 1 
    dv_err = 0;
end

== matlab function land_V0/6DOF-MODEL/动力学/dynamics EQ/MATLAB Function1 ==
  data: phi input; R_bg output; theta input; psi input
function R_bg = ground2body(phi, theta, psi)
T1 = [cos(psi), sin(psi), 0;
     -sin(psi), cos(psi), 0;
      0, 0, 1];
T2 = [cos(theta), 0, -sin(theta);
       0, 1, 0;
      sin(theta), 0, cos(theta)];
T3 = [1, 0, 0;
      0, cos(phi), sin(phi);
      0, -sin(phi), cos(phi)];
R_bg = T3 * T2 * T1;

== matlab function land_V0/6DOF-MODEL/动力学/height/MATLAB Function ==
  data: phi input; R_bg output; theta input; psi input
function R_bg = ground2body(phi, theta, psi)
T1 = [cos(psi), sin(psi), 0;
     -sin(psi), cos(psi), 0;
      0, 0, 1];
T2 = [cos(theta), 0, -sin(theta);
       0, 1, 0;
      sin(theta), 0, cos(theta)];
T3 = [1, 0, 0;
      0, cos(phi), sin(phi);
      0, -sin(phi), cos(phi)];
R_bg = T3 * T2 * T1;

== matlab function land_V0/6DOF-MODEL/动力学/rotation EQ/MATLAB Function1 ==
  data: w input; wB_X output
function wB_X = wB_X(w) 
p = w(1);
q = w(2);
r = w(3);
wB_X = [0, -r,  q;...
        r,  0, -p;...
       -q,  p,  0];

== matlab function land_V0/6DOF-MODEL/动力学/起落架模型/MATLAB Function ==
  data: phi input; R_bg output; theta input; psi input
function R_bg = ground2body(phi, theta, psi)
T1 = [cos(psi), sin(psi), 0;
     -sin(psi), cos(psi), 0;
      0, 0, 1];
T2 = [cos(theta), 0, -sin(theta);
       0, 1, 0;
      sin(theta), 0, cos(theta)];
T3 = [1, 0, 0;
      0, cos(phi), sin(phi);
      0, -sin(phi), cos(phi)];
R_bg = T3 * T2 * T1;

== matlab function land_V0/6DOF-MODEL/动力学/起落架模型/侧向力/Subsystem/MATLAB Function ==
  data: phi input; R_bg output; theta input; psi input
function R_bg = ground2body(phi, theta, psi)
T1 = [cos(psi), sin(psi), 0;
     -sin(psi), cos(psi), 0;
      0, 0, 1];
T2 = [cos(theta), 0, -sin(theta);
       0, 1, 0;
      sin(theta), 0, cos(theta)];
T3 = [1, 0, 0;
      0, cos(phi), sin(phi);
      0, -sin(phi), cos(phi)];
R_bg = T3 * T2 * T1;

== matlab function land_V0/6DOF-MODEL/动力学/起落架模型/侧向力/Subsystem/主轮侧向方向向量 ==
  data: Cbg input; eg_lat output; eb_lat input
function eg_lat = project_main_lat(Cbg, eb_lat)

e_z = [0; 0; 1];              % 前-右-下坐标系：Z 轴向下
P_g = eye(3) - e_z*e_z.';     % 投影到地面水平面

eg_lat = P_g * Cbg * eb_lat;

n = norm(eg_lat);
if n > 1e-8
    eg_lat = eg_lat / n;
else
    eg_lat = [0; 1; 0];       % 默认地面右向
end

== matlab function land_V0/6DOF-MODEL/动力学/起落架模型/侧向力/Subsystem/前轮侧向向量 ==
  data: Cbg input; eg_lat output; eb_lat input
function eg_lat = project_lat(Cbg, eb_lat)

e_z = [0; 0; 1];              % 前-右-下坐标系：Z 轴向下
P_g = eye(3) - e_z*e_z.';     % 投影到地面水平面

eg_lat = P_g * Cbg * eb_lat;

n = norm(eg_lat);
if n > 1e-8
    eg_lat = eg_lat / n;
else
    eg_lat = [0; 1; 0];       % 默认地面右向
end

== matlab function land_V0/6DOF-MODEL/动力学/起落架模型/MATLAB Function1 ==
  data: phi input; R_bg output; theta input; psi input
function R_bg = ground2body(phi, theta, psi)
T1 = [cos(psi), sin(psi), 0;
     -sin(psi), cos(psi), 0;
      0, 0, 1];
T2 = [cos(theta), 0, -sin(theta);
       0, 1, 0;
      sin(theta), 0, cos(theta)];
T3 = [1, 0, 0;
      0, cos(phi), sin(phi);
      0, -sin(phi), cos(phi)];
R_bg = T3 * T2 * T1;

== matlab function land_V0/6DOF-MODEL/动力学/起落架模型/三轮在地系下的力/摩擦圆限幅/前轮摩擦圆限幅 ==
  data: N input; F_long_out output; F_long input; F_lat input; F_lat_out output
function [F_long_out,F_lat_out]=Dround_saturation_nose(N,F_long,F_lat)
mu=0.65;
F_ALL=sqrt((F_long)^2+(F_lat)^2);
if(F_ALL<=mu*N)
    F_long_out=F_long;
    F_lat_out=F_lat;
else
    s=mu*N/F_ALL;
    F_long_out=s*F_long;
    F_lat_out=s*F_lat;
end

== matlab function land_V0/6DOF-MODEL/动力学/起落架模型/三轮在地系下的力/摩擦圆限幅/主轮摩擦圆限幅左 ==
  data: N input; F_long_out output; F_long input; F_lat input; F_lat_out output
function [F_long_out,F_lat_out]=Dround_saturation_main(N,F_long,F_lat)
mu=0.7;
F_ALL=sqrt((F_long)^2+(F_lat)^2);
if(F_ALL<=mu*N)
    F_long_out=F_long;
    F_lat_out=F_lat;
else
    s=mu*N/F_ALL;
    F_long_out=s*F_long;
    F_lat_out=s*F_lat;
end

== matlab function land_V0/6DOF-MODEL/动力学/起落架模型/三轮在地系下的力/摩擦圆限幅/主轮摩擦圆限幅右 ==
  data: N input; F_long_out output; F_long input; F_lat input; F_lat_out output
function [F_long_out,F_lat_out]=Dround_saturation_main(N,F_long,F_lat)
mu=0.7;
F_ALL=sqrt((F_long)^2+(F_lat)^2);
if(F_ALL<=mu*N)
    F_long_out=F_long;
    F_lat_out=F_lat;
else
    s=mu*N/F_ALL;
    F_long_out=s*F_long;
    F_lat_out=s*F_lat;
end

== matlab function land_V0/Guidance/3_空中制导/高度切换/MATLAB Function ==
  data: X input; H_cmd output
function H_cmd = round_H_cmd(X)
%#codegen
% 圆拉平段高度指令
% X: 当前地面坐标 X, m
% H_cmd: 高度指令, m, 向上为正

X_B = -4048.3;
X_C = -3253.6;
X_R = -3044.2;
H_R = 8069.4;
R   = 8000.0;

X_use = X;

if X_use < X_B
    X_use = X_B;
elseif X_use > X_C
    X_use = X_C;
end

dx = X_use - X_R;
rad = R^2 - dx^2;

if rad < 1e-6
    rad = 1e-6;
end

H_cmd = H_R - sqrt(rad);

== matlab function land_V0/6DOF-MODEL/动力学/起落架模型/法向支反力/MATLAB Function ==
  data: phi input; R_bg output; theta input; psi input
function R_bg = ground2body(phi, theta, psi)
T1 = [cos(psi), sin(psi), 0;
     -sin(psi), cos(psi), 0;
      0, 0, 1];
T2 = [cos(theta), 0, -sin(theta);
       0, 1, 0;
      sin(theta), 0, cos(theta)];
T3 = [1, 0, 0;
      0, cos(phi), sin(phi);
      0, -sin(phi), cos(phi)];
R_bg = T3 * T2 * T1;

== matlab function land_V0/Guidance/4_拉平制导/MATLAB Function1 ==
  settings: updateMethod=DISCRETE  sampleTime=0.001
  data: Flight_Phase input; gamma_cmd output; t input; h_AGL input; Vg input
function gamma_cmd = flare_gamma_cmd(Flight_Phase, t, h_AGL, Vg)
%#codegen
% 拉平接地段下滑角指令
%
% Flight_Phase : 当前飞行阶段
% t            : 仿真时间, s
% h_AGL        : 当前离地高度, m，高度向上为正
% Vg           : 地速或水平速度, m/s
% gamma_cmd    : 下滑角指令, rad，下降为负

FLARE_PHASE = 11;     % 如果你的模型用 10 表示拉平接地，就改成 10

T_flare   = 6.0;      % 拉平时间常数, s
V_sink_td = 0.5;      % 期望接地下沉率, m/s

persistent t_enter H_enter last_phase

if isempty(t_enter)
    t_enter = 0.0;
    H_enter = 20.0;
    last_phase = uint8(0);
end

% 进入拉平段瞬间锁存当前高度
if Flight_Phase == FLARE_PHASE && last_phase ~= FLARE_PHASE
    t_enter = t;
    H_enter = h_AGL;

    if H_enter < 0.5
        H_enter = 0.5;
    end
end

if Flight_Phase == FLARE_PHASE
    tau = t - t_enter;

    if tau < 0
        tau = 0;
    end

    H_cmd = (H_enter + V_sink_td * T_flare) * exp(-tau / T_flare) ...
            - V_sink_td * T_flare;

    if H_cmd < 0
        H_cmd = 0;
    end

    Hdot_cmd = -(H_cmd + V_sink_td * T_flare) / T_flare;

    if Vg < 1.0
        Vg = 1.0;
    end

    s = Hdot_cmd / Vg;

    if s > 1.0
        s = 1.0;
    elseif s < -1.0
        s = -1.0;
    end

    gamma_cmd = asin(s);
else
    gamma_cmd = 0.0;
end

last_phase = Flight_Phase;

== matlab function land_V0/6DOF-MODEL/动力学/height/MATLAB Function1 ==
  data: phi input; R_bg output; theta input; psi input
function R_bg = ground2body(phi, theta, psi)
T1 = [cos(psi), sin(psi), 0;
     -sin(psi), cos(psi), 0;
      0, 0, 1];
T2 = [cos(theta), 0, -sin(theta);
       0, 1, 0;
      sin(theta), 0, cos(theta)];
T3 = [1, 0, 0;
      0, cos(phi), sin(phi);
      0, -sin(phi), cos(phi)];
R_bg = T3 * T2 * T1;

== stateflow chart land_V0/Flight Phase Manager/Phase Logic ==
  state Landing_Mode
    state Trajectory_Capture
      en: Flight_Phase = 7;
    state Steep_Glide
      en: Flight_Phase = 8;
    state Approach
      en: Flight_Phase = 6;
    state Flare_Touchdown
      en: Flight_Phase = 11;
    state Shallow_Glide
      en: Flight_Phase = 10;
    state Circular_Flare
      en: Flight_Phase = 9;
    (default) -> Approach
    Approach -> Trajectory_Capture : [Trajectory_capture == true]
    Trajectory_Capture -> Steep_Glide : [In_steep == true]
    Steep_Glide -> Circular_Flare : [In_round == true]
    Shallow_Glide -> Flare_Touchdown : [In_flare == true]
    Circular_Flare -> Shallow_Glide : [In_shallow == true]
  (default) -> (junction 38)
  (junction 38) -> Landing_Mode
  data: Trajectory_capture input; In_steep input; Flight_Phase output uint8 size=1 =0; In_round input; In_shallow input; In_flare input

== matlab function land_V0/6DOF-MODEL/动力学/起落架模型/纵向力/Subsystem/MATLAB Function ==
  data: phi input; R_bg output; theta input; psi input
function R_bg = ground2body(phi, theta, psi)
T1 = [cos(psi), sin(psi), 0;
     -sin(psi), cos(psi), 0;
      0, 0, 1];
T2 = [cos(theta), 0, -sin(theta);
       0, 1, 0;
      sin(theta), 0, cos(theta)];
T3 = [1, 0, 0;
      0, cos(phi), sin(phi);
      0, -sin(phi), cos(phi)];
R_bg = T3 * T2 * T1;

== matlab function land_V0/6DOF-MODEL/动力学/起落架模型/纵向力/Subsystem/主轮滚动方向向量 ==
  data: Cbg input; eg_long output; eb_long input
function eg_long = project_long(Cbg, eb_long)

e_z = [0; 0; 1];              % 前-右-下坐标系：Z 轴向下
P_g = eye(3) - e_z*e_z.';     % 投影到地面水平面

eg_long = P_g * Cbg * eb_long;

n = norm(eg_long);
if n > 1e-8
    eg_long = eg_long / n;
else
    eg_long = [1; 0; 0];
end

== matlab function land_V0/6DOF-MODEL/动力学/起落架模型/纵向力/Subsystem/前轮滚动方向向量 ==
  data: Cbg input; eg_long output; eb_long input
function eg_long = project_long(Cbg, eb_long)

e_z = [0; 0; 1];              % 前-右-下坐标系中，Z 轴为下
P_g = eye(3) - e_z*e_z.';     % 投影到地面水平面

eg_long = P_g * Cbg * eb_long;

n = norm(eg_long);
if n > 1e-8
    eg_long = eg_long / n;
else
    eg_long = [1; 0; 0];
end

== matlab function land_V0/6DOF-MODEL/动力学/起落架模型/起落架三轮质心在地系下位置/MATLAB Function ==
  data: phi input; R_bg output; theta input; psi input
function R_bg = ground2body(phi, theta, psi)
T1 = [cos(psi), sin(psi), 0;
     -sin(psi), cos(psi), 0;
      0, 0, 1];
T2 = [cos(theta), 0, -sin(theta);
       0, 1, 0;
      sin(theta), 0, cos(theta)];
T3 = [1, 0, 0;
      0, cos(phi), sin(phi);
      0, -sin(phi), cos(phi)];
R_bg = T3 * T2 * T1;
